simulink model "stromseitig"  (R2014a)
settings: Solver=ode45  StartTime=0.0  StopTime=10.0  RelTol=1e-3
settings Model: Creator=Hello Cao  LastModifiedBy=Hello Cao
settings HardwareCC: ProdBitPerPointer=64  ProdHWDeviceType=Generic->64-bit Embedded Processor (LLP64)  TargetLongLongMode=on  TargetIntDivRoundTo=Zero  TargetEndianess=LittleEndian  TargetHWDeviceType=MATLAB Host  ProdEqTarget=off

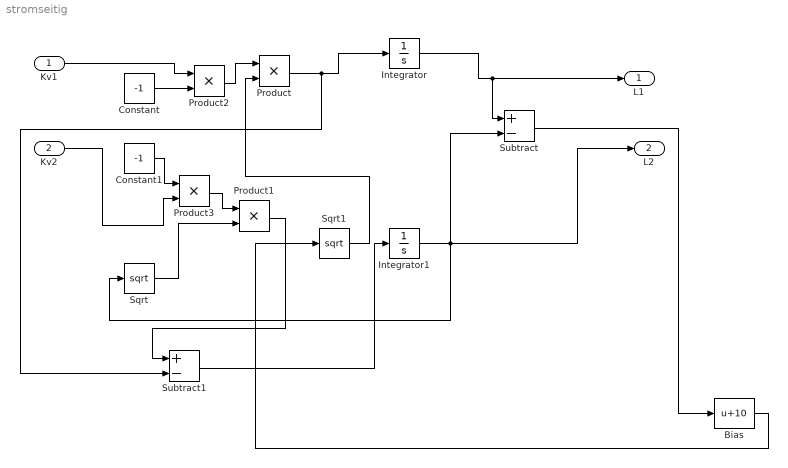
== system stromseitig ==
  Kv1 : Inport
  Kv2 : Inport  Port=2
  Bias : Bias  Bias=10
  Constant : Constant  Value=-1
  Constant1 : Constant  Value=-1
  Integrator : Integrator
  Integrator1 : Integrator
  Product{,1..3} (4 alike) : Product
  Sqrt : Sqrt  SaturateOnIntegerOverflow=on
  Sqrt1 : Sqrt  SaturateOnIntegerOverflow=on
  Subtract : Sum  Inputs=+-
  Subtract1 : Sum  Inputs=+-
  L1 : Outport
  L2 : Outport  Port=2
  wires:
  Kv1/1 -> Product2/1
  Sqrt1/1 -> Product/2
  Product/1 -> Subtract1/2, Integrator/1
  Integrator/1 -> Subtract/1, L1/1
  Kv2/1 -> Product3/2
  Sqrt/1 -> Product1/2
  Integrator1/1 -> Sqrt/1, Subtract/2, L2/1
  Subtract/1 -> Bias/1
  Bias/1 -> Sqrt1/1
  Product1/1 -> Subtract1/1
  Constant/1 -> Product2/2
  Product2/1 -> Product/1
  Constant1/1 -> Product3/1
  Product3/1 -> Product1/1
  Subtract1/1 -> Integrator1/1
